simulink model "four_bit_carry_save_mul_v3"  (R2015a)
settings: Solver=ode45  StartTime=0.0  StopTime=10.0  RelTol=1e-3
libraries: simulink x65
settings Model: CovSFcnEnable=off  Creator=hesham  LastModifiedBy=Ibrah
settings DebuggingCC: SolverPrmCheckMsg=warning

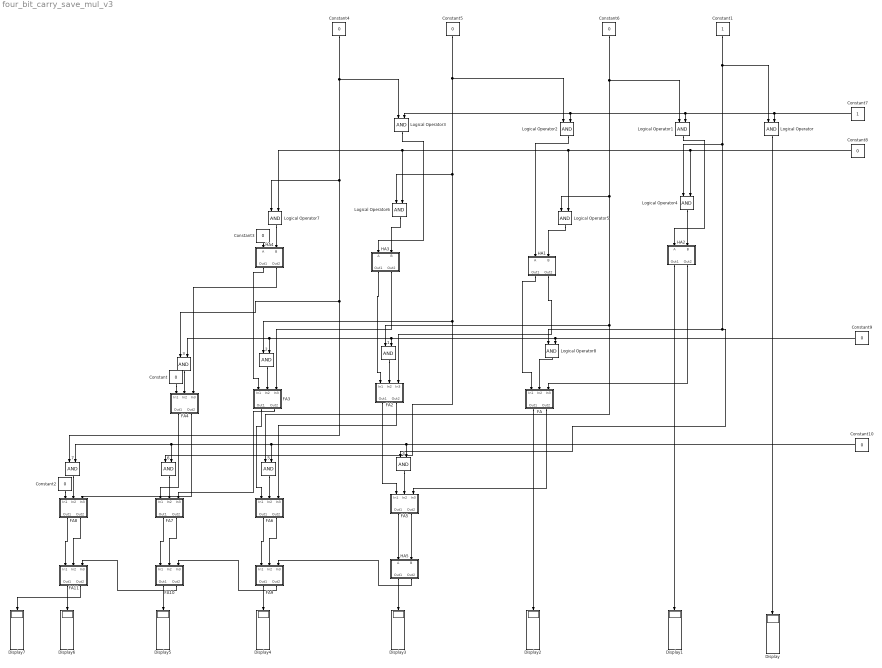
== system four_bit_carry_save_mul_v3 ==
   {1..7} (7 alike) : Logic  AllPortsSameDT=off  OutDataTypeStr=boolean
  Constant{,2..6,8..10} (9 alike) : Constant  Value=0  OutDataTypeStr=boolean
  Constant1 : Constant  OutDataTypeStr=boolean
  Constant7 : Constant  OutDataTypeStr=boolean
  Display{,1..7} (8 alike) : Display
  FA : Subsystem
  FA10 : Subsystem
  FA11 : Subsystem
  FA2 : Subsystem
  FA3 : Subsystem
  FA4 : Subsystem
  FA5 : Subsystem
  FA6 : Subsystem
  FA7 : Subsystem
  FA8 : Subsystem
  FA9 : Subsystem
  HA1 : Subsystem
  HA2 : Subsystem
  HA3 : Subsystem
  HA4 : Subsystem
  HA5 : Subsystem
  Logical Operator{,1..8} (9 alike) : Logic  AllPortsSameDT=off  OutDataTypeStr=boolean
  wires:
  Constant7/1 -> Logical Operator3/2, Logical Operator2/2, Logical Operator1/2, Logical Operator/2
  Constant8/1 -> Logical Operator7/2, Logical Operator6/2, Logical Operator5/2, Logical Operator4/2
  Logical Operator4/1 -> HA2/2(B)
  Logical Operator6/1 -> HA3/2(B)
  Logical Operator5/1 -> HA1/2(B)
  Logical Operator7/1 -> HA4/2(B)
  HA3/1(Out1) -> FA2/1(In1)
  HA4/2(Out2) -> FA4/3(In3)
  HA3/2(Out2) -> FA3/3(In3)
  HA1/2(Out2) -> FA2/3(In3)
  HA2/2(Out2) -> FA/3(In3)
  Constant1/1 -> Logical Operator/1, Logical Operator4/1, " 4"/1, Logical Operator8/1
  Constant6/1 -> " 5"/1, " 1"/1, Logical Operator5/1, Logical Operator1/1
  Constant5/1 -> Logical Operator2/1, Logical Operator6/1, " 6"/1, " 2"/1
  Logical Operator8/1 -> FA/2(In2)
  HA1/1(Out1) -> FA/1(In1)
  Constant9/1 -> " 3"/2, " 2"/2, " 1"/2, Logical Operator8/2
  " 1"/1 -> FA2/2(In2)
  " 2"/1 -> FA3/2(In2)
  " 3"/1 -> FA4/2(In2)
  Constant/1 -> FA4/1(In1)
  HA4/1(Out1) -> FA3/1(In1)
  " 4"/1 -> FA5/2(In2)
  " 5"/1 -> FA6/2(In2)
  " 6"/1 -> FA7/2(In2)
  " 7"/1 -> FA8/2(In2)
  Constant10/1 -> " 7"/2, " 6"/2, " 5"/2, " 4"/2
  Constant4/1 -> Logical Operator3/1, Logical Operator7/1, " 7"/1, " 3"/1
  FA2/1(Out1) -> FA5/1(In1)
  FA3/1(Out1) -> FA6/1(In1)
  FA4/1(Out1) -> FA7/1(In1)
  Constant2/1 -> FA8/1(In1)
  FA/2(Out2) -> FA5/3(In3)
  Constant3/1 -> HA4/1(A)
  Logical Operator3/1 -> HA3/1(A)
  Logical Operator2/1 -> HA1/1(A)
  Logical Operator1/1 -> HA2/1(A)
  HA5/2(Out2) -> FA9/3(In3)
  FA10/2(Out2) -> FA11/3(In3)
  FA2/2(Out2) -> FA6/3(In3)
  FA3/2(Out2) -> FA7/3(In3)
  FA4/2(Out2) -> FA8/3(In3)
  FA5/2(Out2) -> HA5/2(B)
  FA9/2(Out2) -> FA10/3(In3)
  FA11/2(Out2) -> Display7/1
  FA11/1(Out1) -> Display6/1
  FA8/1(Out1) -> FA11/1(In1)
  FA5/1(Out1) -> HA5/1(A)
  FA6/2(Out2) -> FA9/2(In2)
  FA6/1(Out1) -> FA9/1(In1)
  FA7/2(Out2) -> FA10/2(In2)
  FA7/1(Out1) -> FA10/1(In1)
  FA8/2(Out2) -> FA11/2(In2)
  Logical Operator/1 -> Display/1
  HA2/1(Out1) -> Display1/1
  FA/1(Out1) -> Display2/1
  HA5/1(Out1) -> Display3/1
  FA9/1(Out1) -> Display4/1
  FA10/1(Out1) -> Display5/1

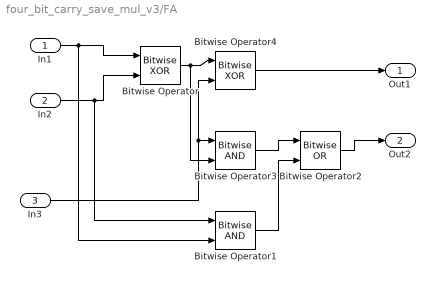
== system four_bit_carry_save_mul_v3/FA ==
  In1 : Inport
  In2 : Inport  Port=2
  In3 : Inport  Port=3
  Bitwise Operator : simulink/Logic and Bit Operations/Bitwise Operator  logicop=XOR  UseBitMask=off  NumInputPorts=2  BitMask=bin2dec('11011001')  BitMaskRealWorld=Stored Integer
  Bitwise Operator1 : simulink/Logic and Bit Operations/Bitwise Operator  logicop=AND  UseBitMask=off  NumInputPorts=2  BitMask=bin2dec('11011001')  BitMaskRealWorld=Stored Integer
  Bitwise Operator2 : simulink/Logic and Bit Operations/Bitwise Operator  logicop=OR  UseBitMask=off  NumInputPorts=2  BitMask=bin2dec('11011001')  BitMaskRealWorld=Stored Integer
  Bitwise Operator3 : simulink/Logic and Bit Operations/Bitwise Operator  logicop=AND  UseBitMask=off  NumInputPorts=2  BitMask=bin2dec('11011001')  BitMaskRealWorld=Stored Integer
  Bitwise Operator4 : simulink/Logic and Bit Operations/Bitwise Operator  logicop=XOR  UseBitMask=off  NumInputPorts=2  BitMask=bin2dec('11011001')  BitMaskRealWorld=Stored Integer
  Out1 : Outport
  Out2 : Outport  Port=2
  wires:
  In1/1 -> Bitwise Operator1/2, Bitwise Operator/1
  In2/1 -> Bitwise Operator1/1, Bitwise Operator/2
  In3/1 -> Bitwise Operator3/1, Bitwise Operator4/2
  Bitwise Operator1/1 -> Bitwise Operator2/2
  Bitwise Operator/1 -> Bitwise Operator3/2, Bitwise Operator4/1
  Bitwise Operator4/1 -> Out1/1
  Bitwise Operator2/1 -> Out2/1
  Bitwise Operator3/1 -> Bitwise Operator2/1

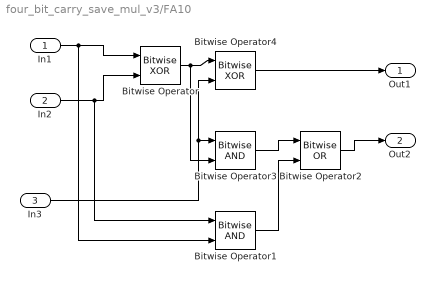
== system four_bit_carry_save_mul_v3/FA10 ==
  In1 : Inport
  In2 : Inport  Port=2
  In3 : Inport  Port=3
  Bitwise Operator : simulink/Logic and Bit Operations/Bitwise Operator  logicop=XOR  UseBitMask=off  NumInputPorts=2  BitMask=bin2dec('11011001')  BitMaskRealWorld=Stored Integer
  Bitwise Operator1 : simulink/Logic and Bit Operations/Bitwise Operator  logicop=AND  UseBitMask=off  NumInputPorts=2  BitMask=bin2dec('11011001')  BitMaskRealWorld=Stored Integer
  Bitwise Operator2 : simulink/Logic and Bit Operations/Bitwise Operator  logicop=OR  UseBitMask=off  NumInputPorts=2  BitMask=bin2dec('11011001')  BitMaskRealWorld=Stored Integer
  Bitwise Operator3 : simulink/Logic and Bit Operations/Bitwise Operator  logicop=AND  UseBitMask=off  NumInputPorts=2  BitMask=bin2dec('11011001')  BitMaskRealWorld=Stored Integer
  Bitwise Operator4 : simulink/Logic and Bit Operations/Bitwise Operator  logicop=XOR  UseBitMask=off  NumInputPorts=2  BitMask=bin2dec('11011001')  BitMaskRealWorld=Stored Integer
  Out1 : Outport
  Out2 : Outport  Port=2
  wires:
  In1/1 -> Bitwise Operator1/2, Bitwise Operator/1
  In2/1 -> Bitwise Operator1/1, Bitwise Operator/2
  In3/1 -> Bitwise Operator3/1, Bitwise Operator4/2
  Bitwise Operator1/1 -> Bitwise Operator2/2
  Bitwise Operator/1 -> Bitwise Operator3/2, Bitwise Operator4/1
  Bitwise Operator4/1 -> Out1/1
  Bitwise Operator2/1 -> Out2/1
  Bitwise Operator3/1 -> Bitwise Operator2/1

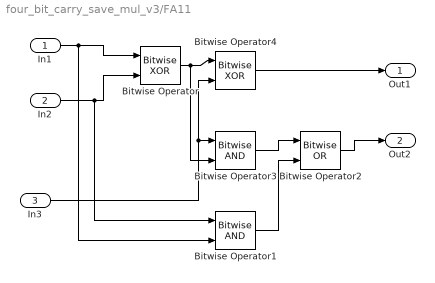
== system four_bit_carry_save_mul_v3/FA11 ==
  In1 : Inport
  In2 : Inport  Port=2
  In3 : Inport  Port=3
  Bitwise Operator : simulink/Logic and Bit Operations/Bitwise Operator  logicop=XOR  UseBitMask=off  NumInputPorts=2  BitMask=bin2dec('11011001')  BitMaskRealWorld=Stored Integer
  Bitwise Operator1 : simulink/Logic and Bit Operations/Bitwise Operator  logicop=AND  UseBitMask=off  NumInputPorts=2  BitMask=bin2dec('11011001')  BitMaskRealWorld=Stored Integer
  Bitwise Operator2 : simulink/Logic and Bit Operations/Bitwise Operator  logicop=OR  UseBitMask=off  NumInputPorts=2  BitMask=bin2dec('11011001')  BitMaskRealWorld=Stored Integer
  Bitwise Operator3 : simulink/Logic and Bit Operations/Bitwise Operator  logicop=AND  UseBitMask=off  NumInputPorts=2  BitMask=bin2dec('11011001')  BitMaskRealWorld=Stored Integer
  Bitwise Operator4 : simulink/Logic and Bit Operations/Bitwise Operator  logicop=XOR  UseBitMask=off  NumInputPorts=2  BitMask=bin2dec('11011001')  BitMaskRealWorld=Stored Integer
  Out1 : Outport
  Out2 : Outport  Port=2
  wires:
  In1/1 -> Bitwise Operator1/2, Bitwise Operator/1
  In2/1 -> Bitwise Operator1/1, Bitwise Operator/2
  In3/1 -> Bitwise Operator3/1, Bitwise Operator4/2
  Bitwise Operator1/1 -> Bitwise Operator2/2
  Bitwise Operator/1 -> Bitwise Operator3/2, Bitwise Operator4/1
  Bitwise Operator4/1 -> Out1/1
  Bitwise Operator2/1 -> Out2/1
  Bitwise Operator3/1 -> Bitwise Operator2/1

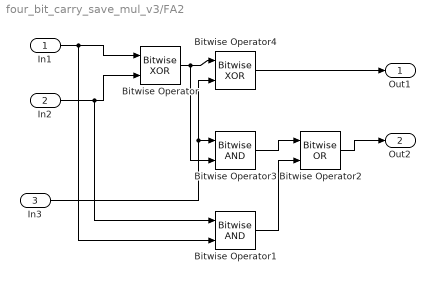
== system four_bit_carry_save_mul_v3/FA2 ==
  In1 : Inport
  In2 : Inport  Port=2
  In3 : Inport  Port=3
  Bitwise Operator : simulink/Logic and Bit Operations/Bitwise Operator  logicop=XOR  UseBitMask=off  NumInputPorts=2  BitMask=bin2dec('11011001')  BitMaskRealWorld=Stored Integer
  Bitwise Operator1 : simulink/Logic and Bit Operations/Bitwise Operator  logicop=AND  UseBitMask=off  NumInputPorts=2  BitMask=bin2dec('11011001')  BitMaskRealWorld=Stored Integer
  Bitwise Operator2 : simulink/Logic and Bit Operations/Bitwise Operator  logicop=OR  UseBitMask=off  NumInputPorts=2  BitMask=bin2dec('11011001')  BitMaskRealWorld=Stored Integer
  Bitwise Operator3 : simulink/Logic and Bit Operations/Bitwise Operator  logicop=AND  UseBitMask=off  NumInputPorts=2  BitMask=bin2dec('11011001')  BitMaskRealWorld=Stored Integer
  Bitwise Operator4 : simulink/Logic and Bit Operations/Bitwise Operator  logicop=XOR  UseBitMask=off  NumInputPorts=2  BitMask=bin2dec('11011001')  BitMaskRealWorld=Stored Integer
  Out1 : Outport
  Out2 : Outport  Port=2
  wires:
  In1/1 -> Bitwise Operator1/2, Bitwise Operator/1
  In2/1 -> Bitwise Operator1/1, Bitwise Operator/2
  In3/1 -> Bitwise Operator3/1, Bitwise Operator4/2
  Bitwise Operator1/1 -> Bitwise Operator2/2
  Bitwise Operator/1 -> Bitwise Operator3/2, Bitwise Operator4/1
  Bitwise Operator4/1 -> Out1/1
  Bitwise Operator2/1 -> Out2/1
  Bitwise Operator3/1 -> Bitwise Operator2/1

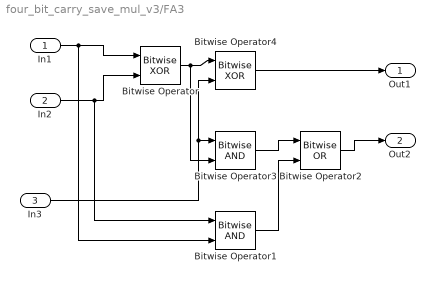
== system four_bit_carry_save_mul_v3/FA3 ==
  In1 : Inport
  In2 : Inport  Port=2
  In3 : Inport  Port=3
  Bitwise Operator : simulink/Logic and Bit Operations/Bitwise Operator  logicop=XOR  UseBitMask=off  NumInputPorts=2  BitMask=bin2dec('11011001')  BitMaskRealWorld=Stored Integer
  Bitwise Operator1 : simulink/Logic and Bit Operations/Bitwise Operator  logicop=AND  UseBitMask=off  NumInputPorts=2  BitMask=bin2dec('11011001')  BitMaskRealWorld=Stored Integer
  Bitwise Operator2 : simulink/Logic and Bit Operations/Bitwise Operator  logicop=OR  UseBitMask=off  NumInputPorts=2  BitMask=bin2dec('11011001')  BitMaskRealWorld=Stored Integer
  Bitwise Operator3 : simulink/Logic and Bit Operations/Bitwise Operator  logicop=AND  UseBitMask=off  NumInputPorts=2  BitMask=bin2dec('11011001')  BitMaskRealWorld=Stored Integer
  Bitwise Operator4 : simulink/Logic and Bit Operations/Bitwise Operator  logicop=XOR  UseBitMask=off  NumInputPorts=2  BitMask=bin2dec('11011001')  BitMaskRealWorld=Stored Integer
  Out1 : Outport
  Out2 : Outport  Port=2
  wires:
  In1/1 -> Bitwise Operator1/2, Bitwise Operator/1
  In2/1 -> Bitwise Operator1/1, Bitwise Operator/2
  In3/1 -> Bitwise Operator3/1, Bitwise Operator4/2
  Bitwise Operator1/1 -> Bitwise Operator2/2
  Bitwise Operator/1 -> Bitwise Operator3/2, Bitwise Operator4/1
  Bitwise Operator4/1 -> Out1/1
  Bitwise Operator2/1 -> Out2/1
  Bitwise Operator3/1 -> Bitwise Operator2/1

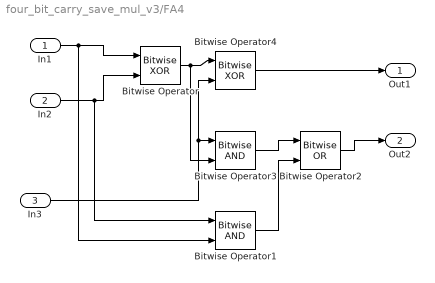
== system four_bit_carry_save_mul_v3/FA4 ==
  In1 : Inport
  In2 : Inport  Port=2
  In3 : Inport  Port=3
  Bitwise Operator : simulink/Logic and Bit Operations/Bitwise Operator  logicop=XOR  UseBitMask=off  NumInputPorts=2  BitMask=bin2dec('11011001')  BitMaskRealWorld=Stored Integer
  Bitwise Operator1 : simulink/Logic and Bit Operations/Bitwise Operator  logicop=AND  UseBitMask=off  NumInputPorts=2  BitMask=bin2dec('11011001')  BitMaskRealWorld=Stored Integer
  Bitwise Operator2 : simulink/Logic and Bit Operations/Bitwise Operator  logicop=OR  UseBitMask=off  NumInputPorts=2  BitMask=bin2dec('11011001')  BitMaskRealWorld=Stored Integer
  Bitwise Operator3 : simulink/Logic and Bit Operations/Bitwise Operator  logicop=AND  UseBitMask=off  NumInputPorts=2  BitMask=bin2dec('11011001')  BitMaskRealWorld=Stored Integer
  Bitwise Operator4 : simulink/Logic and Bit Operations/Bitwise Operator  logicop=XOR  UseBitMask=off  NumInputPorts=2  BitMask=bin2dec('11011001')  BitMaskRealWorld=Stored Integer
  Out1 : Outport
  Out2 : Outport  Port=2
  wires:
  In1/1 -> Bitwise Operator1/2, Bitwise Operator/1
  In2/1 -> Bitwise Operator1/1, Bitwise Operator/2
  In3/1 -> Bitwise Operator3/1, Bitwise Operator4/2
  Bitwise Operator1/1 -> Bitwise Operator2/2
  Bitwise Operator/1 -> Bitwise Operator3/2, Bitwise Operator4/1
  Bitwise Operator4/1 -> Out1/1
  Bitwise Operator2/1 -> Out2/1
  Bitwise Operator3/1 -> Bitwise Operator2/1

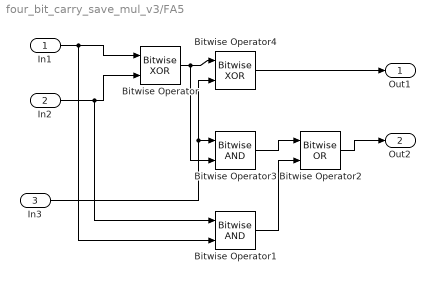
== system four_bit_carry_save_mul_v3/FA5 ==
  In1 : Inport
  In2 : Inport  Port=2
  In3 : Inport  Port=3
  Bitwise Operator : simulink/Logic and Bit Operations/Bitwise Operator  logicop=XOR  UseBitMask=off  NumInputPorts=2  BitMask=bin2dec('11011001')  BitMaskRealWorld=Stored Integer
  Bitwise Operator1 : simulink/Logic and Bit Operations/Bitwise Operator  logicop=AND  UseBitMask=off  NumInputPorts=2  BitMask=bin2dec('11011001')  BitMaskRealWorld=Stored Integer
  Bitwise Operator2 : simulink/Logic and Bit Operations/Bitwise Operator  logicop=OR  UseBitMask=off  NumInputPorts=2  BitMask=bin2dec('11011001')  BitMaskRealWorld=Stored Integer
  Bitwise Operator3 : simulink/Logic and Bit Operations/Bitwise Operator  logicop=AND  UseBitMask=off  NumInputPorts=2  BitMask=bin2dec('11011001')  BitMaskRealWorld=Stored Integer
  Bitwise Operator4 : simulink/Logic and Bit Operations/Bitwise Operator  logicop=XOR  UseBitMask=off  NumInputPorts=2  BitMask=bin2dec('11011001')  BitMaskRealWorld=Stored Integer
  Out1 : Outport
  Out2 : Outport  Port=2
  wires:
  In1/1 -> Bitwise Operator1/2, Bitwise Operator/1
  In2/1 -> Bitwise Operator1/1, Bitwise Operator/2
  In3/1 -> Bitwise Operator3/1, Bitwise Operator4/2
  Bitwise Operator1/1 -> Bitwise Operator2/2
  Bitwise Operator/1 -> Bitwise Operator3/2, Bitwise Operator4/1
  Bitwise Operator4/1 -> Out1/1
  Bitwise Operator2/1 -> Out2/1
  Bitwise Operator3/1 -> Bitwise Operator2/1

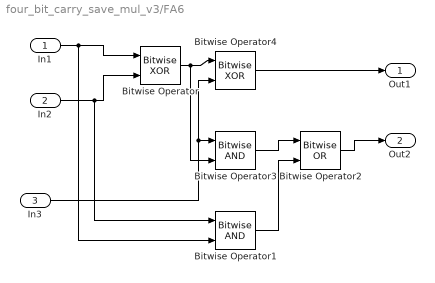
== system four_bit_carry_save_mul_v3/FA6 ==
  In1 : Inport
  In2 : Inport  Port=2
  In3 : Inport  Port=3
  Bitwise Operator : simulink/Logic and Bit Operations/Bitwise Operator  logicop=XOR  UseBitMask=off  NumInputPorts=2  BitMask=bin2dec('11011001')  BitMaskRealWorld=Stored Integer
  Bitwise Operator1 : simulink/Logic and Bit Operations/Bitwise Operator  logicop=AND  UseBitMask=off  NumInputPorts=2  BitMask=bin2dec('11011001')  BitMaskRealWorld=Stored Integer
  Bitwise Operator2 : simulink/Logic and Bit Operations/Bitwise Operator  logicop=OR  UseBitMask=off  NumInputPorts=2  BitMask=bin2dec('11011001')  BitMaskRealWorld=Stored Integer
  Bitwise Operator3 : simulink/Logic and Bit Operations/Bitwise Operator  logicop=AND  UseBitMask=off  NumInputPorts=2  BitMask=bin2dec('11011001')  BitMaskRealWorld=Stored Integer
  Bitwise Operator4 : simulink/Logic and Bit Operations/Bitwise Operator  logicop=XOR  UseBitMask=off  NumInputPorts=2  BitMask=bin2dec('11011001')  BitMaskRealWorld=Stored Integer
  Out1 : Outport
  Out2 : Outport  Port=2
  wires:
  In1/1 -> Bitwise Operator1/2, Bitwise Operator/1
  In2/1 -> Bitwise Operator1/1, Bitwise Operator/2
  In3/1 -> Bitwise Operator3/1, Bitwise Operator4/2
  Bitwise Operator1/1 -> Bitwise Operator2/2
  Bitwise Operator/1 -> Bitwise Operator3/2, Bitwise Operator4/1
  Bitwise Operator4/1 -> Out1/1
  Bitwise Operator2/1 -> Out2/1
  Bitwise Operator3/1 -> Bitwise Operator2/1

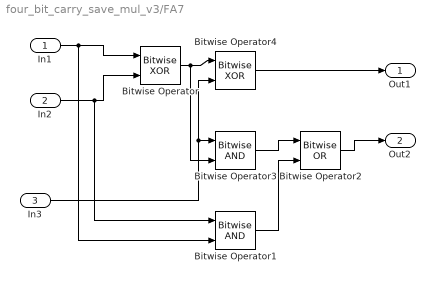
== system four_bit_carry_save_mul_v3/FA7 ==
  In1 : Inport
  In2 : Inport  Port=2
  In3 : Inport  Port=3
  Bitwise Operator : simulink/Logic and Bit Operations/Bitwise Operator  logicop=XOR  UseBitMask=off  NumInputPorts=2  BitMask=bin2dec('11011001')  BitMaskRealWorld=Stored Integer
  Bitwise Operator1 : simulink/Logic and Bit Operations/Bitwise Operator  logicop=AND  UseBitMask=off  NumInputPorts=2  BitMask=bin2dec('11011001')  BitMaskRealWorld=Stored Integer
  Bitwise Operator2 : simulink/Logic and Bit Operations/Bitwise Operator  logicop=OR  UseBitMask=off  NumInputPorts=2  BitMask=bin2dec('11011001')  BitMaskRealWorld=Stored Integer
  Bitwise Operator3 : simulink/Logic and Bit Operations/Bitwise Operator  logicop=AND  UseBitMask=off  NumInputPorts=2  BitMask=bin2dec('11011001')  BitMaskRealWorld=Stored Integer
  Bitwise Operator4 : simulink/Logic and Bit Operations/Bitwise Operator  logicop=XOR  UseBitMask=off  NumInputPorts=2  BitMask=bin2dec('11011001')  BitMaskRealWorld=Stored Integer
  Out1 : Outport
  Out2 : Outport  Port=2
  wires:
  In1/1 -> Bitwise Operator1/2, Bitwise Operator/1
  In2/1 -> Bitwise Operator1/1, Bitwise Operator/2
  In3/1 -> Bitwise Operator3/1, Bitwise Operator4/2
  Bitwise Operator1/1 -> Bitwise Operator2/2
  Bitwise Operator/1 -> Bitwise Operator3/2, Bitwise Operator4/1
  Bitwise Operator4/1 -> Out1/1
  Bitwise Operator2/1 -> Out2/1
  Bitwise Operator3/1 -> Bitwise Operator2/1

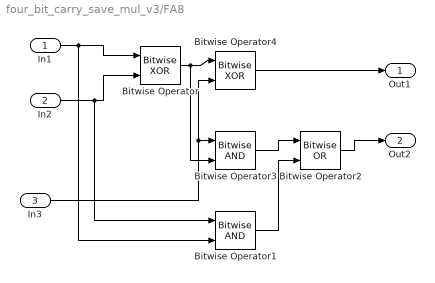
== system four_bit_carry_save_mul_v3/FA8 ==
  In1 : Inport
  In2 : Inport  Port=2
  In3 : Inport  Port=3
  Bitwise Operator : simulink/Logic and Bit Operations/Bitwise Operator  logicop=XOR  UseBitMask=off  NumInputPorts=2  BitMask=bin2dec('11011001')  BitMaskRealWorld=Stored Integer
  Bitwise Operator1 : simulink/Logic and Bit Operations/Bitwise Operator  logicop=AND  UseBitMask=off  NumInputPorts=2  BitMask=bin2dec('11011001')  BitMaskRealWorld=Stored Integer
  Bitwise Operator2 : simulink/Logic and Bit Operations/Bitwise Operator  logicop=OR  UseBitMask=off  NumInputPorts=2  BitMask=bin2dec('11011001')  BitMaskRealWorld=Stored Integer
  Bitwise Operator3 : simulink/Logic and Bit Operations/Bitwise Operator  logicop=AND  UseBitMask=off  NumInputPorts=2  BitMask=bin2dec('11011001')  BitMaskRealWorld=Stored Integer
  Bitwise Operator4 : simulink/Logic and Bit Operations/Bitwise Operator  logicop=XOR  UseBitMask=off  NumInputPorts=2  BitMask=bin2dec('11011001')  BitMaskRealWorld=Stored Integer
  Out1 : Outport
  Out2 : Outport  Port=2
  wires:
  In1/1 -> Bitwise Operator1/2, Bitwise Operator/1
  In2/1 -> Bitwise Operator1/1, Bitwise Operator/2
  In3/1 -> Bitwise Operator3/1, Bitwise Operator4/2
  Bitwise Operator1/1 -> Bitwise Operator2/2
  Bitwise Operator/1 -> Bitwise Operator3/2, Bitwise Operator4/1
  Bitwise Operator4/1 -> Out1/1
  Bitwise Operator2/1 -> Out2/1
  Bitwise Operator3/1 -> Bitwise Operator2/1

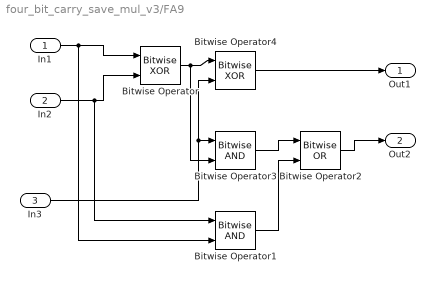
== system four_bit_carry_save_mul_v3/FA9 ==
  In1 : Inport
  In2 : Inport  Port=2
  In3 : Inport  Port=3
  Bitwise Operator : simulink/Logic and Bit Operations/Bitwise Operator  logicop=XOR  UseBitMask=off  NumInputPorts=2  BitMask=bin2dec('11011001')  BitMaskRealWorld=Stored Integer
  Bitwise Operator1 : simulink/Logic and Bit Operations/Bitwise Operator  logicop=AND  UseBitMask=off  NumInputPorts=2  BitMask=bin2dec('11011001')  BitMaskRealWorld=Stored Integer
  Bitwise Operator2 : simulink/Logic and Bit Operations/Bitwise Operator  logicop=OR  UseBitMask=off  NumInputPorts=2  BitMask=bin2dec('11011001')  BitMaskRealWorld=Stored Integer
  Bitwise Operator3 : simulink/Logic and Bit Operations/Bitwise Operator  logicop=AND  UseBitMask=off  NumInputPorts=2  BitMask=bin2dec('11011001')  BitMaskRealWorld=Stored Integer
  Bitwise Operator4 : simulink/Logic and Bit Operations/Bitwise Operator  logicop=XOR  UseBitMask=off  NumInputPorts=2  BitMask=bin2dec('11011001')  BitMaskRealWorld=Stored Integer
  Out1 : Outport
  Out2 : Outport  Port=2
  wires:
  In1/1 -> Bitwise Operator1/2, Bitwise Operator/1
  In2/1 -> Bitwise Operator1/1, Bitwise Operator/2
  In3/1 -> Bitwise Operator3/1, Bitwise Operator4/2
  Bitwise Operator1/1 -> Bitwise Operator2/2
  Bitwise Operator/1 -> Bitwise Operator3/2, Bitwise Operator4/1
  Bitwise Operator4/1 -> Out1/1
  Bitwise Operator2/1 -> Out2/1
  Bitwise Operator3/1 -> Bitwise Operator2/1

== system four_bit_carry_save_mul_v3/HA1 ==
  note: HA
  A : Inport
  B : Inport  Port=2
  Bitwise Operator : simulink/Logic and Bit Operations/Bitwise Operator  logicop=XOR  UseBitMask=off  NumInputPorts=2  BitMask=bin2dec('11011001')  BitMaskRealWorld=Stored Integer
  Bitwise Operator1 : simulink/Logic and Bit Operations/Bitwise Operator  logicop=AND  UseBitMask=off  NumInputPorts=2  BitMask=bin2dec('11011001')  BitMaskRealWorld=Stored Integer
  Out1 : Outport
  Out2 : Outport  Port=2
  wires:
  A/1 -> Bitwise Operator1/2, Bitwise Operator/1
  B/1 -> Bitwise Operator1/1, Bitwise Operator/2
  Bitwise Operator1/1 -> Out2/1
  Bitwise Operator/1 -> Out1/1

== system four_bit_carry_save_mul_v3/HA2 ==
  note: HA
  A : Inport
  B : Inport  Port=2
  Bitwise Operator : simulink/Logic and Bit Operations/Bitwise Operator  logicop=XOR  UseBitMask=off  NumInputPorts=2  BitMask=bin2dec('11011001')  BitMaskRealWorld=Stored Integer
  Bitwise Operator1 : simulink/Logic and Bit Operations/Bitwise Operator  logicop=AND  UseBitMask=off  NumInputPorts=2  BitMask=bin2dec('11011001')  BitMaskRealWorld=Stored Integer
  Out1 : Outport
  Out2 : Outport  Port=2
  wires:
  A/1 -> Bitwise Operator1/2, Bitwise Operator/1
  B/1 -> Bitwise Operator1/1, Bitwise Operator/2
  Bitwise Operator1/1 -> Out2/1
  Bitwise Operator/1 -> Out1/1

== system four_bit_carry_save_mul_v3/HA3 ==
  note: HA
  A : Inport
  B : Inport  Port=2
  Bitwise Operator : simulink/Logic and Bit Operations/Bitwise Operator  logicop=XOR  UseBitMask=off  NumInputPorts=2  BitMask=bin2dec('11011001')  BitMaskRealWorld=Stored Integer
  Bitwise Operator1 : simulink/Logic and Bit Operations/Bitwise Operator  logicop=AND  UseBitMask=off  NumInputPorts=2  BitMask=bin2dec('11011001')  BitMaskRealWorld=Stored Integer
  Out1 : Outport
  Out2 : Outport  Port=2
  wires:
  A/1 -> Bitwise Operator1/2, Bitwise Operator/1
  B/1 -> Bitwise Operator1/1, Bitwise Operator/2
  Bitwise Operator1/1 -> Out2/1
  Bitwise Operator/1 -> Out1/1

== system four_bit_carry_save_mul_v3/HA4 ==
  note: HA
  A : Inport
  B : Inport  Port=2
  Bitwise Operator : simulink/Logic and Bit Operations/Bitwise Operator  logicop=XOR  UseBitMask=off  NumInputPorts=2  BitMask=bin2dec('11011001')  BitMaskRealWorld=Stored Integer
  Bitwise Operator1 : simulink/Logic and Bit Operations/Bitwise Operator  logicop=AND  UseBitMask=off  NumInputPorts=2  BitMask=bin2dec('11011001')  BitMaskRealWorld=Stored Integer
  Out1 : Outport
  Out2 : Outport  Port=2
  wires:
  A/1 -> Bitwise Operator1/2, Bitwise Operator/1
  B/1 -> Bitwise Operator1/1, Bitwise Operator/2
  Bitwise Operator1/1 -> Out2/1
  Bitwise Operator/1 -> Out1/1

== system four_bit_carry_save_mul_v3/HA5 ==
  note: HA
  A : Inport
  B : Inport  Port=2
  Bitwise Operator : simulink/Logic and Bit Operations/Bitwise Operator  logicop=XOR  UseBitMask=off  NumInputPorts=2  BitMask=bin2dec('11011001')  BitMaskRealWorld=Stored Integer
  Bitwise Operator1 : simulink/Logic and Bit Operations/Bitwise Operator  logicop=AND  UseBitMask=off  NumInputPorts=2  BitMask=bin2dec('11011001')  BitMaskRealWorld=Stored Integer
  Out1 : Outport
  Out2 : Outport  Port=2
  wires:
  A/1 -> Bitwise Operator1/2, Bitwise Operator/1
  B/1 -> Bitwise Operator1/1, Bitwise Operator/2
  Bitwise Operator1/1 -> Out2/1
  Bitwise Operator/1 -> Out1/1
